simulink model "IEEE39_11gen"  (R2020a)
settings: Solver=FixedStepAuto  StartTime=0  StopTime=5  FixedStep=Ts  RelTol=1e-3
values from neighbouring files (symbols this model uses):
  Ts = 1/Fs    [ModifiedIEEE39_11gen.m]
  Wbase = Fbase*2*pi    [ModifiedIEEE39_11gen.m]
  Ybase = 1/Zbase    [ModifiedIEEE39_11gen.m]
  Zbase = Vbase/Ibase    [ModifiedIEEE39_11gen.m]
undefined symbols (not defined in the file or in its folder): ApparatusDiscreDamping, ApparatusPara, ApparatusPowerFlow, ApparatusType, OtherInputs, PowerFlow, x_e
libraries: powerlib x131, SimplusGT x51
settings Model: Creator=Qiufan_Yang  LastModifiedBy=Qiufan_Yang

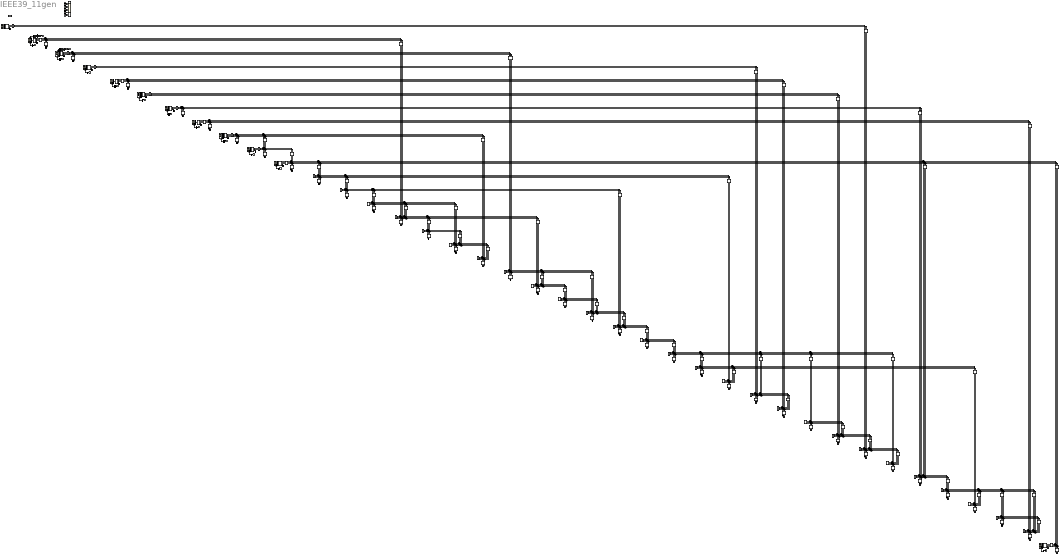
== system IEEE39_11gen ==
  B-GND{2,4,7,10,12,14,17,19,23,26,29,32,35,37,39..40,43,45,47,49,51,53,58,61..62,64..65,67,69,71..72,74,78..79,81..82} (36 alike) : powerlib/Elements/Ground  LConnTagsString=a
  Branch1-32 : powerlib/Elements/Three-Phase Series RLC Branch  LConnTagsString=A|B|C  RConnTagsString=A|B|C  BranchType=L  Resistance=(0)*Zbase  Inductance=(0.016321)*Zbase/Wbase  Capacitance=1e-6  Measurements=None
  Branch10-10 : powerlib/Elements/Three-Phase Parallel RLC Branch  LConnTagsString=A|B|C  RConnTagsString=A|B|C  BranchType=C  Resistance=(Inf)*Zbase  Inductance=(Inf)*Zbase/Wbase  Capacitance=(0.05)*Ybase/Wbase  Measurements=None
      settings: SourceProductBaseCode=PS
  Branch10-11 : powerlib/Elements/Three-Phase Series RLC Branch  LConnTagsString=A|B|C  RConnTagsString=A|B|C  BranchType=L  Resistance=(0)*Zbase  Inductance=(0.024661)*Zbase/Wbase  Capacitance=1e-6  Measurements=None
  Branch11-11 : powerlib/Elements/Three-Phase Parallel RLC Branch  LConnTagsString=A|B|C  RConnTagsString=A|B|C  BranchType=C  Resistance=(Inf)*Zbase  Inductance=(Inf)*Zbase/Wbase  Capacitance=(0.05)*Ybase/Wbase  Measurements=None
      settings: SourceProductBaseCode=PS
  Branch11-12 : powerlib/Elements/Three-Phase Series RLC Branch  LConnTagsString=A|B|C  RConnTagsString=A|B|C  BranchType=L  Resistance=(0)*Zbase  Inductance=(0.0090596)*Zbase/Wbase  Capacitance=1e-6  Measurements=None
  Branch11-34 : powerlib/Elements/Three-Phase Series RLC Branch  LConnTagsString=A|B|C  RConnTagsString=A|B|C  BranchType=L  Resistance=(0)*Zbase  Inductance=(0.00516)*Zbase/Wbase  Capacitance=1e-6  Measurements=None
  Branch11-39 : powerlib/Elements/Three-Phase Series RLC Branch  LConnTagsString=A|B|C  RConnTagsString=A|B|C  BranchType=L  Resistance=(0)*Zbase  Inductance=(0.01086)*Zbase/Wbase  Capacitance=1e-6  Measurements=None
  Branch12-12 : powerlib/Elements/Three-Phase Parallel RLC Branch  LConnTagsString=A|B|C  RConnTagsString=A|B|C  BranchType=C  Resistance=(Inf)*Zbase  Inductance=(Inf)*Zbase/Wbase  Capacitance=(0.03)*Ybase/Wbase  Measurements=None
      settings: SourceProductBaseCode=PS
  Branch12-13 : powerlib/Elements/Three-Phase Series RLC Branch  LConnTagsString=A|B|C  RConnTagsString=A|B|C  BranchType=L  Resistance=(0)*Zbase  Inductance=(0.01278)*Zbase/Wbase  Capacitance=1e-6  Measurements=None
  Branch12-27 : powerlib/Elements/Three-Phase Series RLC Branch  LConnTagsString=A|B|C  RConnTagsString=A|B|C  BranchType=L  Resistance=(0)*Zbase  Inductance=(0.0079802)*Zbase/Wbase  Capacitance=1e-6  Measurements=None
  Branch13-13 : powerlib/Elements/Three-Phase Parallel RLC Branch  LConnTagsString=A|B|C  RConnTagsString=A|B|C  BranchType=C  Resistance=(Inf)*Zbase  Inductance=(Inf)*Zbase/Wbase  Capacitance=(0.03)*Ybase/Wbase  Measurements=None
      settings: SourceProductBaseCode=PS
  Branch13-14 : powerlib/Elements/Three-Phase Series RLC Branch  LConnTagsString=A|B|C  RConnTagsString=A|B|C  BranchType=L  Resistance=(0)*Zbase  Inductance=(0.0076799)*Zbase/Wbase  Capacitance=1e-6  Measurements=None
  Branch13-23 : powerlib/Elements/Three-Phase Series RLC Branch  LConnTagsString=A|B|C  RConnTagsString=A|B|C  BranchType=L  Resistance=(0)*Zbase  Inductance=(0.0077399)*Zbase/Wbase  Capacitance=1e-6  Measurements=None
  Branch14-14 : powerlib/Elements/Three-Phase Parallel RLC Branch  LConnTagsString=A|B|C  RConnTagsString=A|B|C  BranchType=C  Resistance=(Inf)*Zbase  Inductance=(Inf)*Zbase/Wbase  Capacitance=(0.03)*Ybase/Wbase  Measurements=None
      settings: SourceProductBaseCode=PS
  Branch14-15 : powerlib/Elements/Three-Phase Series RLC Branch  LConnTagsString=A|B|C  RConnTagsString=A|B|C  BranchType=L  Resistance=(0)*Zbase  Inductance=(0.00156)*Zbase/Wbase  Capacitance=1e-6  Measurements=None
  Branch14-17 : powerlib/Elements/Three-Phase Series RLC Branch  LConnTagsString=A|B|C  RConnTagsString=A|B|C  BranchType=L  Resistance=(0)*Zbase  Inductance=(0.00672)*Zbase/Wbase  Capacitance=1e-6  Measurements=None
  Branch15-15 : powerlib/Elements/Three-Phase Parallel RLC Branch  LConnTagsString=A|B|C  RConnTagsString=A|B|C  BranchType=C  Resistance=(Inf)*Zbase  Inductance=(Inf)*Zbase/Wbase  Capacitance=(0.03)*Ybase/Wbase  Measurements=None
      settings: SourceProductBaseCode=PS
  Branch15-16 : powerlib/Elements/Three-Phase Series RLC Branch  LConnTagsString=A|B|C  RConnTagsString=A|B|C  BranchType=L  Resistance=(0)*Zbase  Inductance=(0.00552)*Zbase/Wbase  Capacitance=1e-6  Measurements=None
  Branch15-20 : powerlib/Elements/Three-Phase Series RLC Branch  LConnTagsString=A|B|C  RConnTagsString=A|B|C  BranchType=L  Resistance=(0)*Zbase  Inductance=(0.00492)*Zbase/Wbase  Capacitance=1e-6  Measurements=None
  Branch16-16 : powerlib/Elements/Three-Phase Parallel RLC Branch  LConnTagsString=A|B|C  RConnTagsString=A|B|C  BranchType=C  Resistance=(Inf)*Zbase  Inductance=(Inf)*Zbase/Wbase  Capacitance=(0.03)*Ybase/Wbase  Measurements=None
      settings: SourceProductBaseCode=PS
  Branch16-17 : powerlib/Elements/Three-Phase Series RLC Branch  LConnTagsString=A|B|C  RConnTagsString=A|B|C  BranchType=L  Resistance=(0)*Zbase  Inductance=(0.00276)*Zbase/Wbase  Capacitance=1e-6  Measurements=None
  Branch17-17 : powerlib/Elements/Three-Phase Parallel RLC Branch  LConnTagsString=A|B|C  RConnTagsString=A|B|C  BranchType=C  Resistance=(Inf)*Zbase  Inductance=(Inf)*Zbase/Wbase  Capacitance=(0.03)*Ybase/Wbase  Measurements=None
      settings: SourceProductBaseCode=PS
  Branch17-18 : powerlib/Elements/Three-Phase Series RLC Branch  LConnTagsString=A|B|C  RConnTagsString=A|B|C  BranchType=L  Resistance=(0)*Zbase  Inductance=(0.021782)*Zbase/Wbase  Capacitance=1e-6  Measurements=None
  Branch18-18 : powerlib/Elements/Three-Phase Parallel RLC Branch  LConnTagsString=A|B|C  RConnTagsString=A|B|C  BranchType=C  Resistance=(Inf)*Zbase  Inductance=(Inf)*Zbase/Wbase  Capacitance=(0.03)*Ybase/Wbase  Measurements=None
      settings: SourceProductBaseCode=PS
  Branch19-19 : powerlib/Elements/Three-Phase Parallel RLC Branch  LConnTagsString=A|B|C  RConnTagsString=A|B|C  BranchType=C  Resistance=(Inf)*Zbase  Inductance=(Inf)*Zbase/Wbase  Capacitance=(0.03)*Ybase/Wbase  Measurements=None
      settings: SourceProductBaseCode=PS
  Branch19-20 : powerlib/Elements/Three-Phase Series RLC Branch  LConnTagsString=A|B|C  RConnTagsString=A|B|C  BranchType=L  Resistance=(0)*Zbase  Inductance=(0.00258)*Zbase/Wbase  Capacitance=1e-6  Measurements=None
  Branch19-22 : powerlib/Elements/Three-Phase Series RLC Branch  LConnTagsString=A|B|C  RConnTagsString=A|B|C  BranchType=L  Resistance=(0)*Zbase  Inductance=(0.00258)*Zbase/Wbase  Capacitance=1e-6  Measurements=None
  Branch2-15 : powerlib/Elements/Three-Phase Series RLC Branch  LConnTagsString=A|B|C  RConnTagsString=A|B|C  BranchType=L  Resistance=(0)*Zbase  Inductance=(0.014999)*Zbase/Wbase  Capacitance=1e-6  Measurements=None
  Branch2-2 : powerlib/Elements/Three-Phase Parallel RLC Branch  LConnTagsString=A|B|C  RConnTagsString=A|B|C  BranchType=C  Resistance=(Inf)*Zbase  Inductance=(Inf)*Zbase/Wbase  Capacitance=(0.05)*Ybase/Wbase  Measurements=None
      settings: SourceProductBaseCode=PS
  Branch20-20 : powerlib/Elements/Three-Phase Parallel RLC Branch  LConnTagsString=A|B|C  RConnTagsString=A|B|C  BranchType=C  Resistance=(Inf)*Zbase  Inductance=(Inf)*Zbase/Wbase  Capacitance=(0.03)*Ybase/Wbase  Measurements=None
      settings: SourceProductBaseCode=PS
  Branch20-21 : powerlib/Elements/Three-Phase Series RLC Branch  LConnTagsString=A|B|C  RConnTagsString=A|B|C  BranchType=L  Resistance=(0)*Zbase  Inductance=(0.026103)*Zbase/Wbase  Capacitance=1e-6  Measurements=None
  Branch21-21 : powerlib/Elements/Three-Phase Parallel RLC Branch  LConnTagsString=A|B|C  RConnTagsString=A|B|C  BranchType=C  Resistance=(Inf)*Zbase  Inductance=(Inf)*Zbase/Wbase  Capacitance=(0.03)*Ybase/Wbase  Measurements=None
      settings: SourceProductBaseCode=PS
  Branch21-22 : powerlib/Elements/Three-Phase Series RLC Branch  LConnTagsString=A|B|C  RConnTagsString=A|B|C  BranchType=L  Resistance=(0)*Zbase  Inductance=(0.026103)*Zbase/Wbase  Capacitance=1e-6  Measurements=None
  Branch22-22 : powerlib/Elements/Three-Phase Parallel RLC Branch  LConnTagsString=A|B|C  RConnTagsString=A|B|C  BranchType=C  Resistance=(Inf)*Zbase  Inductance=(Inf)*Zbase/Wbase  Capacitance=(0.03)*Ybase/Wbase  Measurements=None
      settings: SourceProductBaseCode=PS
  Branch22-23 : powerlib/Elements/Three-Phase Series RLC Branch  LConnTagsString=A|B|C  RConnTagsString=A|B|C  BranchType=L  Resistance=(0)*Zbase  Inductance=(0.0060599)*Zbase/Wbase  Capacitance=1e-6  Measurements=None
  Branch23-23 : powerlib/Elements/Three-Phase Parallel RLC Branch  LConnTagsString=A|B|C  RConnTagsString=A|B|C  BranchType=C  Resistance=(Inf)*Zbase  Inductance=(Inf)*Zbase/Wbase  Capacitance=(0.03)*Ybase/Wbase  Measurements=None
      settings: SourceProductBaseCode=PS
  Branch23-24 : powerlib/Elements/Three-Phase Series RLC Branch  LConnTagsString=A|B|C  RConnTagsString=A|B|C  BranchType=L  Resistance=(0)*Zbase  Inductance=(0.013021)*Zbase/Wbase  Capacitance=1e-6  Measurements=None
  Branch24-24 : powerlib/Elements/Three-Phase Parallel RLC Branch  LConnTagsString=A|B|C  RConnTagsString=A|B|C  BranchType=C  Resistance=(Inf)*Zbase  Inductance=(Inf)*Zbase/Wbase  Capacitance=(0.03)*Ybase/Wbase  Measurements=None
      settings: SourceProductBaseCode=PS
  Branch24-25 : powerlib/Elements/Three-Phase Series RLC Branch  LConnTagsString=A|B|C  RConnTagsString=A|B|C  BranchType=L  Resistance=(0)*Zbase  Inductance=(0.0056398)*Zbase/Wbase  Capacitance=1e-6  Measurements=None
  Branch25-25 : powerlib/Elements/Three-Phase Parallel RLC Branch  LConnTagsString=A|B|C  RConnTagsString=A|B|C  BranchType=C  Resistance=(Inf)*Zbase  Inductance=(Inf)*Zbase/Wbase  Capacitance=(0.03)*Ybase/Wbase  Measurements=None
      settings: SourceProductBaseCode=PS
  Branch25-26 : powerlib/Elements/Three-Phase Series RLC Branch  LConnTagsString=A|B|C  RConnTagsString=A|B|C  BranchType=L  Resistance=(0)*Zbase  Inductance=(0.0053399)*Zbase/Wbase  Capacitance=1e-6  Measurements=None
  Branch25-28 : powerlib/Elements/Three-Phase Series RLC Branch  LConnTagsString=A|B|C  RConnTagsString=A|B|C  BranchType=L  Resistance=(0)*Zbase  Inductance=(0.0117)*Zbase/Wbase  Capacitance=1e-6  Measurements=None
  Branch25-30 : powerlib/Elements/Three-Phase Series RLC Branch  LConnTagsString=A|B|C  RConnTagsString=A|B|C  BranchType=L  Resistance=(0)*Zbase  Inductance=(0.0080998)*Zbase/Wbase  Capacitance=1e-6  Measurements=None
  Branch25-33 : powerlib/Elements/Three-Phase Series RLC Branch  LConnTagsString=A|B|C  RConnTagsString=A|B|C  BranchType=L  Resistance=(0)*Zbase  Inductance=(0.0035399)*Zbase/Wbase  Capacitance=1e-6  Measurements=None
  Branch26-26 : powerlib/Elements/Three-Phase Parallel RLC Branch  LConnTagsString=A|B|C  RConnTagsString=A|B|C  BranchType=C  Resistance=(Inf)*Zbase  Inductance=(Inf)*Zbase/Wbase  Capacitance=(0.03)*Ybase/Wbase  Measurements=None
      settings: SourceProductBaseCode=PS
  Branch26-27 : powerlib/Elements/Three-Phase Series RLC Branch  LConnTagsString=A|B|C  RConnTagsString=A|B|C  BranchType=L  Resistance=(0)*Zbase  Inductance=(0.00492)*Zbase/Wbase  Capacitance=1e-6  Measurements=None
  Branch26-36 : powerlib/Elements/Three-Phase Series RLC Branch  LConnTagsString=A|B|C  RConnTagsString=A|B|C  BranchType=L  Resistance=(0)*Zbase  Inductance=(0.01038)*Zbase/Wbase  Capacitance=1e-6  Measurements=None
  Branch27-27 : powerlib/Elements/Three-Phase Parallel RLC Branch  LConnTagsString=A|B|C  RConnTagsString=A|B|C  BranchType=C  Resistance=(Inf)*Zbase  Inductance=(Inf)*Zbase/Wbase  Capacitance=(0.03)*Ybase/Wbase  Measurements=None
      settings: SourceProductBaseCode=PS
  Branch28-28 : powerlib/Elements/Three-Phase Parallel RLC Branch  LConnTagsString=A|B|C  RConnTagsString=A|B|C  BranchType=C  Resistance=(Inf)*Zbase  Inductance=(Inf)*Zbase/Wbase  Capacitance=(0.03)*Ybase/Wbase  Measurements=None
      settings: SourceProductBaseCode=PS
  Branch28-29 : powerlib/Elements/Three-Phase Series RLC Branch  LConnTagsString=A|B|C  RConnTagsString=A|B|C  BranchType=L  Resistance=(0)*Zbase  Inductance=(0.0082802)*Zbase/Wbase  Capacitance=1e-6  Measurements=None
  Branch29-29 : powerlib/Elements/Three-Phase Parallel RLC Branch  LConnTagsString=A|B|C  RConnTagsString=A|B|C  BranchType=C  Resistance=(Inf)*Zbase  Inductance=(Inf)*Zbase/Wbase  Capacitance=(0.03)*Ybase/Wbase  Measurements=None
      settings: SourceProductBaseCode=PS
  Branch3-19 : powerlib/Elements/Three-Phase Series RLC Branch  LConnTagsString=A|B|C  RConnTagsString=A|B|C  BranchType=L  Resistance=(0)*Zbase  Inductance=(0.012)*Zbase/Wbase  Capacitance=1e-6  Measurements=None
  Branch3-3 : powerlib/Elements/Three-Phase Parallel RLC Branch  LConnTagsString=A|B|C  RConnTagsString=A|B|C  BranchType=C  Resistance=(Inf)*Zbase  Inductance=(Inf)*Zbase/Wbase  Capacitance=(0.05)*Ybase/Wbase  Measurements=None
      settings: SourceProductBaseCode=PS
  Branch30-30 : powerlib/Elements/Three-Phase Parallel RLC Branch  LConnTagsString=A|B|C  RConnTagsString=A|B|C  BranchType=C  Resistance=(Inf)*Zbase  Inductance=(Inf)*Zbase/Wbase  Capacitance=(0.03)*Ybase/Wbase  Measurements=None
      settings: SourceProductBaseCode=PS
  Branch30-31 : powerlib/Elements/Three-Phase Series RLC Branch  LConnTagsString=A|B|C  RConnTagsString=A|B|C  BranchType=L  Resistance=(0)*Zbase  Inductance=(0.0083998)*Zbase/Wbase  Capacitance=1e-6  Measurements=None
  Branch31-31 : powerlib/Elements/Three-Phase Parallel RLC Branch  LConnTagsString=A|B|C  RConnTagsString=A|B|C  BranchType=C  Resistance=(Inf)*Zbase  Inductance=(Inf)*Zbase/Wbase  Capacitance=(0.03)*Ybase/Wbase  Measurements=None
      settings: SourceProductBaseCode=PS
  Branch31-32 : powerlib/Elements/Three-Phase Series RLC Branch  LConnTagsString=A|B|C  RConnTagsString=A|B|C  BranchType=L  Resistance=(0)*Zbase  Inductance=(0.00576)*Zbase/Wbase  Capacitance=1e-6  Measurements=None
  Branch32-32 : powerlib/Elements/Three-Phase Parallel RLC Branch  LConnTagsString=A|B|C  RConnTagsString=A|B|C  BranchType=C  Resistance=(Inf)*Zbase  Inductance=(Inf)*Zbase/Wbase  Capacitance=(0.03)*Ybase/Wbase  Measurements=None
      settings: SourceProductBaseCode=PS
  Branch32-33 : powerlib/Elements/Three-Phase Series RLC Branch  LConnTagsString=A|B|C  RConnTagsString=A|B|C  BranchType=L  Resistance=(0)*Zbase  Inductance=(0.021)*Zbase/Wbase  Capacitance=1e-6  Measurements=None
  Branch33-33 : powerlib/Elements/Three-Phase Parallel RLC Branch  LConnTagsString=A|B|C  RConnTagsString=A|B|C  BranchType=C  Resistance=(Inf)*Zbase  Inductance=(Inf)*Zbase/Wbase  Capacitance=(0.03)*Ybase/Wbase  Measurements=None
      settings: SourceProductBaseCode=PS
  Branch34-34 : powerlib/Elements/Three-Phase Parallel RLC Branch  LConnTagsString=A|B|C  RConnTagsString=A|B|C  BranchType=C  Resistance=(Inf)*Zbase  Inductance=(Inf)*Zbase/Wbase  Capacitance=(0.03)*Ybase/Wbase  Measurements=None
      settings: SourceProductBaseCode=PS
  Branch34-35 : powerlib/Elements/Three-Phase Series RLC Branch  LConnTagsString=A|B|C  RConnTagsString=A|B|C  BranchType=L  Resistance=(0)*Zbase  Inductance=(0.019011)*Zbase/Wbase  Capacitance=1e-6  Measurements=None
  Branch35-35 : powerlib/Elements/Three-Phase Parallel RLC Branch  LConnTagsString=A|B|C  RConnTagsString=A|B|C  BranchType=C  Resistance=(Inf)*Zbase  Inductance=(Inf)*Zbase/Wbase  Capacitance=(0.03)*Ybase/Wbase  Measurements=None
      settings: SourceProductBaseCode=PS
  Branch35-36 : powerlib/Elements/Three-Phase Series RLC Branch  LConnTagsString=A|B|C  RConnTagsString=A|B|C  BranchType=L  Resistance=(0)*Zbase  Inductance=(0.0088199)*Zbase/Wbase  Capacitance=1e-6  Measurements=None
  Branch35-37 : powerlib/Elements/Three-Phase Series RLC Branch  LConnTagsString=A|B|C  RConnTagsString=A|B|C  BranchType=L  Resistance=(0)*Zbase  Inductance=(0.028441)*Zbase/Wbase  Capacitance=1e-6  Measurements=None
  Branch35-38 : powerlib/Elements/Three-Phase Series RLC Branch  LConnTagsString=A|B|C  RConnTagsString=A|B|C  BranchType=L  Resistance=(0)*Zbase  Inductance=(0.037495)*Zbase/Wbase  Capacitance=1e-6  Measurements=None
  Branch36-36 : powerlib/Elements/Three-Phase Parallel RLC Branch  LConnTagsString=A|B|C  RConnTagsString=A|B|C  BranchType=C  Resistance=(Inf)*Zbase  Inductance=(Inf)*Zbase/Wbase  Capacitance=(0.03)*Ybase/Wbase  Measurements=None
      settings: SourceProductBaseCode=PS
  Branch37-37 : powerlib/Elements/Three-Phase Parallel RLC Branch  LConnTagsString=A|B|C  RConnTagsString=A|B|C  BranchType=C  Resistance=(Inf)*Zbase  Inductance=(Inf)*Zbase/Wbase  Capacitance=(0.03)*Ybase/Wbase  Measurements=None
      settings: SourceProductBaseCode=PS
  Branch37-38 : powerlib/Elements/Three-Phase Series RLC Branch  LConnTagsString=A|B|C  RConnTagsString=A|B|C  BranchType=L  Resistance=(0)*Zbase  Inductance=(0.0090596)*Zbase/Wbase  Capacitance=1e-6  Measurements=None
  Branch38-38 : powerlib/Elements/Three-Phase Parallel RLC Branch  LConnTagsString=A|B|C  RConnTagsString=A|B|C  BranchType=C  Resistance=(Inf)*Zbase  Inductance=(Inf)*Zbase/Wbase  Capacitance=(0.03)*Ybase/Wbase  Measurements=None
      settings: SourceProductBaseCode=PS
  Branch39-39 : powerlib/Elements/Three-Phase Parallel RLC Branch  LConnTagsString=A|B|C  RConnTagsString=A|B|C  BranchType=C  Resistance=(Inf)*Zbase  Inductance=(Inf)*Zbase/Wbase  Capacitance=(0.05)*Ybase/Wbase  Measurements=None
      settings: SourceProductBaseCode=PS
  Branch4-28 : powerlib/Elements/Three-Phase Series RLC Branch  LConnTagsString=A|B|C  RConnTagsString=A|B|C  BranchType=L  Resistance=(0)*Zbase  Inductance=(0.0085201)*Zbase/Wbase  Capacitance=1e-6  Measurements=None
  Branch5-29 : powerlib/Elements/Three-Phase Series RLC Branch  LConnTagsString=A|B|C  RConnTagsString=A|B|C  BranchType=L  Resistance=(0)*Zbase  Inductance=(0.0108)*Zbase/Wbase  Capacitance=1e-6  Measurements=None
  Branch5-5 : powerlib/Elements/Three-Phase Parallel RLC Branch  LConnTagsString=A|B|C  RConnTagsString=A|B|C  BranchType=C  Resistance=(Inf)*Zbase  Inductance=(Inf)*Zbase/Wbase  Capacitance=(0.05)*Ybase/Wbase  Measurements=None
      settings: SourceProductBaseCode=PS
  Branch6-31 : powerlib/Elements/Three-Phase Series RLC Branch  LConnTagsString=A|B|C  RConnTagsString=A|B|C  BranchType=L  Resistance=(0)*Zbase  Inductance=(0.00858)*Zbase/Wbase  Capacitance=1e-6  Measurements=None
  Branch7-34 : powerlib/Elements/Three-Phase Series RLC Branch  LConnTagsString=A|B|C  RConnTagsString=A|B|C  BranchType=L  Resistance=(0)*Zbase  Inductance=(0.01392)*Zbase/Wbase  Capacitance=1e-6  Measurements=None
  Branch7-7 : powerlib/Elements/Three-Phase Parallel RLC Branch  LConnTagsString=A|B|C  RConnTagsString=A|B|C  BranchType=C  Resistance=(Inf)*Zbase  Inductance=(Inf)*Zbase/Wbase  Capacitance=(0.05)*Ybase/Wbase  Measurements=None
      settings: SourceProductBaseCode=PS
  Branch8-38 : powerlib/Elements/Three-Phase Series RLC Branch  LConnTagsString=A|B|C  RConnTagsString=A|B|C  BranchType=L  Resistance=(0)*Zbase  Inductance=(0.0093598)*Zbase/Wbase  Capacitance=1e-6  Measurements=None
  Branch8-8 : powerlib/Elements/Three-Phase Parallel RLC Branch  LConnTagsString=A|B|C  RConnTagsString=A|B|C  BranchType=C  Resistance=(Inf)*Zbase  Inductance=(Inf)*Zbase/Wbase  Capacitance=(0.05)*Ybase/Wbase  Measurements=None
      settings: SourceProductBaseCode=PS
  Branch9-10 : powerlib/Elements/Three-Phase Series RLC Branch  LConnTagsString=A|B|C  RConnTagsString=A|B|C  BranchType=L  Resistance=(0)*Zbase  Inductance=(0.014999)*Zbase/Wbase  Capacitance=1e-6  Measurements=None
  Branch9-18 : powerlib/Elements/Three-Phase Series RLC Branch  LConnTagsString=A|B|C  RConnTagsString=A|B|C  BranchType=L  Resistance=(0)*Zbase  Inductance=(0.014999)*Zbase/Wbase  Capacitance=1e-6  Measurements=None
  Branch9-9 : powerlib/Elements/Three-Phase Parallel RLC Branch  LConnTagsString=A|B|C  RConnTagsString=A|B|C  BranchType=C  Resistance=(Inf)*Zbase  Inductance=(Inf)*Zbase/Wbase  Capacitance=(0.05)*Ybase/Wbase  Measurements=None
      settings: SourceProductBaseCode=PS
  Bus{1..39} (39 alike) : SimplusGT/Three-Phase Bus  Vbase=1  Sbase=1
      settings: SourceProductName=Simplus Grid Tool
  D-GND{1..11,39} (12 alike) : powerlib/Elements/Ground  LConnTagsString=a
  D-Scope{1..11,39} (12 alike) : Scope  NumInputPorts=7
  DS-Bus{1..11,39} (12 alike) : BusSelector  OutputSignals=v_dq,i_dq,v_abc,i_abc,w,theta,pq
  Demux{1..13} (13 alike) : Demux  Outputs=2
  Inf-Bus1 : SimplusGT/AC Infinite Bus (Voltage Type)  Ts=Ts  Sbase=Sbase  Vbase=Vbase  Wbase=Wbase  vd=PowerFlow{1}(3)  vq=0  theta0=PowerFlow{1}(4)  w=Wbase  R=1e-30
      settings: SourceProductName=Simplus Grid Tool
  Scope1 : Scope  NumInputPorts=9
  Sqrt1 : Sqrt  SaturateOnIntegerOverflow=on
  Sqrt2 : Sqrt  SaturateOnIntegerOverflow=on
  Square{2..5} (4 alike) : Math  Operator=square  SaturateOnIntegerOverflow=on
  Sum1 : Sum  Inputs=|++
  Sum2 : Sum  Inputs=|++
  VSI-Droop4 : SimplusGT/Grid-Forming Voltage-Source Inverter (dq-Frame System Object)  Ts=Ts  Sbase=Sbase  Vbase=Vbase  Wbase=Wbase  ApparatusType=ApparatusType{4}  ApparatusPara=ApparatusPara{4}  PowerFlow=ApparatusPowerFlow{4}  x0=x_e{4}  OtherInputs=OtherInputs{4}  DiscreMethod=Hybrid Trapezoidal  EnableInsideModification=off  DiscreDampingFlag=on  DiscreDampingValue=ApparatusDiscreDamping{4}  LinearizationTimes=1  DirectFeedthrough=off
      settings: SourceProductName=Simplus Grid Tool
  VSI-Droop6 : SimplusGT/Grid-Forming Voltage-Source Inverter (dq-Frame System Object)  Ts=Ts  Sbase=Sbase  Vbase=Vbase  Wbase=Wbase  ApparatusType=ApparatusType{6}  ApparatusPara=ApparatusPara{6}  PowerFlow=ApparatusPowerFlow{6}  x0=x_e{6}  OtherInputs=OtherInputs{6}  DiscreMethod=Hybrid Trapezoidal  EnableInsideModification=off  DiscreDampingFlag=on  DiscreDampingValue=ApparatusDiscreDamping{6}  LinearizationTimes=1  DirectFeedthrough=off
      settings: SourceProductName=Simplus Grid Tool
  VSI-PLL10 : SimplusGT/Grid-Following Voltage-Source Inverter (dq-Frame System Object)  Ts=Ts  Sbase=Sbase  Vbase=Vbase  Wbase=Wbase  ApparatusType=ApparatusType{10}  ApparatusPara=ApparatusPara{10}  PowerFlow=ApparatusPowerFlow{10}  x0=x_e{10}  OtherInputs=OtherInputs{10}  DiscreMethod=Hybrid Trapezoidal  EnableInsideModification=off  DiscreDampingFlag=on  DiscreDampingValue=ApparatusDiscreDamping{10}  LinearizationTimes=1  DirectFeedthrough=off
      settings: SourceProductName=Simplus Grid Tool
  VSI-PLL11 : SimplusGT/Grid-Following Voltage-Source Inverter (dq-Frame System Object)  Ts=Ts  Sbase=Sbase  Vbase=Vbase  Wbase=Wbase  ApparatusType=ApparatusType{11}  ApparatusPara=ApparatusPara{11}  PowerFlow=ApparatusPowerFlow{11}  x0=x_e{11}  OtherInputs=OtherInputs{11}  DiscreMethod=Hybrid Trapezoidal  EnableInsideModification=off  DiscreDampingFlag=on  DiscreDampingValue=ApparatusDiscreDamping{11}  LinearizationTimes=1  DirectFeedthrough=off
      settings: SourceProductName=Simplus Grid Tool
  VSI-PLL2 : SimplusGT/Grid-Following Voltage-Source Inverter (dq-Frame System Object)  Ts=Ts  Sbase=Sbase  Vbase=Vbase  Wbase=Wbase  ApparatusType=ApparatusType{2}  ApparatusPara=ApparatusPara{2}  PowerFlow=ApparatusPowerFlow{2}  x0=x_e{2}  OtherInputs=OtherInputs{2}  DiscreMethod=Hybrid Trapezoidal  EnableInsideModification=off  DiscreDampingFlag=on  DiscreDampingValue=ApparatusDiscreDamping{2}  LinearizationTimes=1  DirectFeedthrough=off
      settings: SourceProductName=Simplus Grid Tool
  VSI-PLL3 : SimplusGT/Grid-Following Voltage-Source Inverter (dq-Frame System Object)  Ts=Ts  Sbase=Sbase  Vbase=Vbase  Wbase=Wbase  ApparatusType=ApparatusType{3}  ApparatusPara=ApparatusPara{3}  PowerFlow=ApparatusPowerFlow{3}  x0=x_e{3}  OtherInputs=OtherInputs{3}  DiscreMethod=Hybrid Trapezoidal  EnableInsideModification=off  DiscreDampingFlag=on  DiscreDampingValue=ApparatusDiscreDamping{3}  LinearizationTimes=1  DirectFeedthrough=off
      settings: SourceProductName=Simplus Grid Tool
  VSI-PLL39 : SimplusGT/Grid-Following Voltage-Source Inverter (dq-Frame System Object)  Ts=Ts  Sbase=Sbase  Vbase=Vbase  Wbase=Wbase  ApparatusType=ApparatusType{39}  ApparatusPara=ApparatusPara{39}  PowerFlow=ApparatusPowerFlow{39}  x0=x_e{39}  OtherInputs=OtherInputs{39}  DiscreMethod=Hybrid Trapezoidal  EnableInsideModification=off  DiscreDampingFlag=on  DiscreDampingValue=ApparatusDiscreDamping{39}  LinearizationTimes=1  DirectFeedthrough=off
      settings: SourceProductName=Simplus Grid Tool
  VSI-PLL5 : SimplusGT/Grid-Following Voltage-Source Inverter (dq-Frame System Object)  Ts=Ts  Sbase=Sbase  Vbase=Vbase  Wbase=Wbase  ApparatusType=ApparatusType{5}  ApparatusPara=ApparatusPara{5}  PowerFlow=ApparatusPowerFlow{5}  x0=x_e{5}  OtherInputs=OtherInputs{5}  DiscreMethod=Hybrid Trapezoidal  EnableInsideModification=off  DiscreDampingFlag=on  DiscreDampingValue=ApparatusDiscreDamping{5}  LinearizationTimes=1  DirectFeedthrough=off
      settings: SourceProductName=Simplus Grid Tool
  VSI-PLL7 : SimplusGT/Grid-Following Voltage-Source Inverter (dq-Frame System Object)  Ts=Ts  Sbase=Sbase  Vbase=Vbase  Wbase=Wbase  ApparatusType=ApparatusType{7}  ApparatusPara=ApparatusPara{7}  PowerFlow=ApparatusPowerFlow{7}  x0=x_e{7}  OtherInputs=OtherInputs{7}  DiscreMethod=Hybrid Trapezoidal  EnableInsideModification=off  DiscreDampingFlag=on  DiscreDampingValue=ApparatusDiscreDamping{7}  LinearizationTimes=1  DirectFeedthrough=off
      settings: SourceProductName=Simplus Grid Tool
  VSI-PLL8 : SimplusGT/Grid-Following Voltage-Source Inverter (dq-Frame System Object)  Ts=Ts  Sbase=Sbase  Vbase=Vbase  Wbase=Wbase  ApparatusType=ApparatusType{8}  ApparatusPara=ApparatusPara{8}  PowerFlow=ApparatusPowerFlow{8}  x0=x_e{8}  OtherInputs=OtherInputs{8}  DiscreMethod=Hybrid Trapezoidal  EnableInsideModification=off  DiscreDampingFlag=on  DiscreDampingValue=ApparatusDiscreDamping{8}  LinearizationTimes=1  DirectFeedthrough=off
      settings: SourceProductName=Simplus Grid Tool
  VSI-PLL9 : SimplusGT/Grid-Following Voltage-Source Inverter (dq-Frame System Object)  Ts=Ts  Sbase=Sbase  Vbase=Vbase  Wbase=Wbase  ApparatusType=ApparatusType{9}  ApparatusPara=ApparatusPara{9}  PowerFlow=ApparatusPowerFlow{9}  x0=x_e{9}  OtherInputs=OtherInputs{9}  DiscreMethod=Hybrid Trapezoidal  EnableInsideModification=off  DiscreDampingFlag=on  DiscreDampingValue=ApparatusDiscreDamping{9}  LinearizationTimes=1  DirectFeedthrough=off
      settings: SourceProductName=Simplus Grid Tool
  powergui : powerlib/powergui  Priority=1  SimulationMode=Discrete  SampleTime=Ts  frequency=60  Iterations=50  frequencyindice=0  Pbase=100e6  ErrMax=1e-4  UnitsV=kV  UnitsW=MW  buscounter=0  FunctionMessages=off  echomessages=off  EnableUseOfTLC=off  CurrentSourceSwitches=off  DisableSnubberDevices=off  DisableRonSwitches=off  DisableVfSwitches=off  DisplayEquations=off  AutomaticDiscreteSolvers=off  SolverType=Tustin/Backward Euler (TBE)  Interpol=off  ExternalGateDelay=off  methode=off  Ts=100  x0status=blocks  SPID=on  SwTol=0  HookPort=off  NonlinearTolerance=1e-4  nMaxIteration=100  ContinueOnMaxIteration=off  RestoreLinks=warning  ResistiveCurrentMeasurement=off  Frange=[0:2:500]  Ylog=off  Xlog=on  ShowGrid=off  save=off  variable=ZData  structure=0  ZoomFFT=off  StartTime=0.0  cycles=1  DisplayStyle=1  fundamental=60  FreqAxis=off  MaxFrequency=1000  frequencyindicesteady=1  RmsSteady=1  display=off
  wires:
  Inf-Bus1/1 -> DS-Bus1/1
  DS-Bus1/1 -> D-Scope1/1  "<v_dq>"
  DS-Bus1/2 -> D-Scope1/2  "<i_dq>"
  DS-Bus1/3 -> D-Scope1/3  "<v_abc>"
  DS-Bus1/4 -> D-Scope1/4  "<i_abc>"
  DS-Bus1/5 -> D-Scope1/5  "<w>"
  DS-Bus1/6 -> D-Scope1/6  "<theta>"
  DS-Bus1/7 -> D-Scope1/7  "<pq>"
  VSI-PLL2/1 -> DS-Bus2/1
  DS-Bus2/2 -> D-Scope2/2  "<i_dq>"
  DS-Bus2/3 -> D-Scope2/3  "<v_abc>"
  DS-Bus2/4 -> D-Scope2/4  "<i_abc>"
  DS-Bus2/5 -> D-Scope2/5  "<w>"
  DS-Bus2/6 -> D-Scope2/6  "<theta>"
  VSI-PLL3/1 -> DS-Bus3/1
  DS-Bus3/2 -> D-Scope3/2  "<i_dq>"
  DS-Bus3/3 -> D-Scope3/3  "<v_abc>"
  DS-Bus3/4 -> D-Scope3/4  "<i_abc>"
  DS-Bus3/5 -> D-Scope3/5  "<w>"
  DS-Bus3/6 -> D-Scope3/6  "<theta>"
  VSI-Droop4/1 -> DS-Bus4/1
  DS-Bus4/1 -> D-Scope4/1  "<v_dq>"
  DS-Bus4/2 -> D-Scope4/2  "<i_dq>"
  DS-Bus4/3 -> D-Scope4/3  "<v_abc>"
  DS-Bus4/4 -> D-Scope4/4  "<i_abc>"
  DS-Bus4/5 -> D-Scope4/5  "<w>"
  DS-Bus4/6 -> D-Scope4/6  "<theta>"
  VSI-PLL5/1 -> DS-Bus5/1
  DS-Bus5/1 -> D-Scope5/1  "<v_dq>"
  DS-Bus5/2 -> D-Scope5/2  "<i_dq>"
  DS-Bus5/3 -> D-Scope5/3  "<v_abc>"
  DS-Bus5/4 -> D-Scope5/4  "<i_abc>"
  DS-Bus5/5 -> D-Scope5/5  "<w>"
  DS-Bus5/6 -> D-Scope5/6  "<theta>"
  VSI-Droop6/1 -> DS-Bus6/1
  DS-Bus6/1 -> D-Scope6/1  "<v_dq>"
  DS-Bus6/2 -> D-Scope6/2  "<i_dq>"
  DS-Bus6/3 -> D-Scope6/3  "<v_abc>"
  DS-Bus6/4 -> D-Scope6/4  "<i_abc>"
  DS-Bus6/5 -> D-Scope6/5  "<w>"
  DS-Bus6/6 -> D-Scope6/6  "<theta>"
  VSI-PLL7/1 -> DS-Bus7/1
  DS-Bus7/1 -> D-Scope7/1  "<v_dq>"
  DS-Bus7/2 -> D-Scope7/2  "<i_dq>"
  DS-Bus7/3 -> D-Scope7/3  "<v_abc>"
  DS-Bus7/4 -> D-Scope7/4  "<i_abc>"
  DS-Bus7/5 -> D-Scope7/5  "<w>"
  DS-Bus7/6 -> D-Scope7/6  "<theta>"
  VSI-PLL8/1 -> DS-Bus8/1
  DS-Bus8/1 -> D-Scope8/1  "<v_dq>"
  DS-Bus8/2 -> D-Scope8/2  "<i_dq>"
  DS-Bus8/3 -> D-Scope8/3  "<v_abc>"
  DS-Bus8/4 -> D-Scope8/4  "<i_abc>"
  DS-Bus8/5 -> D-Scope8/5  "<w>"
  DS-Bus8/6 -> D-Scope8/6  "<theta>"
  VSI-PLL9/1 -> DS-Bus9/1
  DS-Bus9/1 -> D-Scope9/1  "<v_dq>"
  DS-Bus9/2 -> D-Scope9/2  "<i_dq>"
  DS-Bus9/3 -> D-Scope9/3  "<v_abc>"
  DS-Bus9/4 -> D-Scope9/4  "<i_abc>"
  DS-Bus9/5 -> D-Scope9/5  "<w>"
  DS-Bus9/6 -> D-Scope9/6  "<theta>"
  VSI-PLL10/1 -> DS-Bus10/1
  DS-Bus10/1 -> D-Scope10/1  "<v_dq>"
  DS-Bus10/2 -> D-Scope10/2  "<i_dq>"
  DS-Bus10/3 -> D-Scope10/3  "<v_abc>"
  DS-Bus10/4 -> D-Scope10/4  "<i_abc>"
  DS-Bus10/5 -> D-Scope10/5  "<w>"
  DS-Bus10/6 -> D-Scope10/6  "<theta>"
  VSI-PLL11/1 -> DS-Bus11/1
  DS-Bus11/1 -> D-Scope11/1  "<v_dq>"
  DS-Bus11/2 -> D-Scope11/2  "<i_dq>"
  DS-Bus11/3 -> D-Scope11/3  "<v_abc>"
  DS-Bus11/4 -> D-Scope11/4  "<i_abc>"
  DS-Bus11/5 -> D-Scope11/5  "<w>"
  DS-Bus11/6 -> D-Scope11/6  "<theta>"
  VSI-PLL39/1 -> DS-Bus39/1
  DS-Bus39/1 -> D-Scope39/1  "<v_dq>"
  DS-Bus39/2 -> D-Scope39/2  "<i_dq>"
  DS-Bus39/3 -> D-Scope39/3  "<v_abc>"
  DS-Bus39/4 -> D-Scope39/4  "<i_abc>"
  DS-Bus39/5 -> D-Scope39/5  "<w>"
  DS-Bus39/6 -> D-Scope39/6  "<theta>"
  Demux1/1 -> Square2/1
  Square2/1 -> Sum1/1
  DS-Bus2/1 -> Demux1/1, D-Scope2/1  "<v_dq>"
  Sqrt1/1 -> [u2]
  Sum1/1 -> Sqrt1/1
  Square3/1 -> Sum1/2
  Demux1/2 -> Square3/1
  DS-Bus3/1 -> Demux2/1, D-Scope3/1  "<v_dq>"
  Square5/1 -> Sum2/2
  Sqrt2/1 -> [u3]
  Square4/1 -> Sum2/1
  Demux2/2 -> Square5/1
  Demux2/1 -> Square4/1
  Sum2/1 -> Sqrt2/1
  Demux11/1 -> [p2]
  DS-Bus2/7 -> Demux11/1, D-Scope2/7  "<pq>"
  Demux3/1 -> [p3]
  DS-Bus3/7 -> Demux3/1, D-Scope3/7  "<pq>"
  Demux4/1 -> [p4]
  DS-Bus4/7 -> Demux4/1, D-Scope4/7  "<pq>"
  Demux5/1 -> [p5]
  DS-Bus5/7 -> Demux5/1, D-Scope5/7  "<pq>"
  Demux6/1 -> [p6]
  DS-Bus6/7 -> Demux6/1, D-Scope6/7  "<pq>"
  Demux7/1 -> [p7]
  DS-Bus7/7 -> Demux7/1, D-Scope7/7  "<pq>"
  Demux8/1 -> [p8]
  DS-Bus8/7 -> Demux8/1, D-Scope8/7  "<pq>"
  Demux9/1 -> [p9]
  DS-Bus9/7 -> Demux9/1, D-Scope9/7  "<pq>"
  Demux10/1 -> [p10]
  DS-Bus10/7 -> Demux10/1, D-Scope10/7  "<pq>"
  Demux12/1 -> [p11]
  DS-Bus11/7 -> Demux12/1, D-Scope11/7  "<pq>"
  Demux13/1 -> [p1]
  DS-Bus39/7 -> Demux13/1, D-Scope39/7  "<pq>"
  [p2] -> Scope1/2
  [p9] -> Scope1/7
  [p7] -> Scope1/5
  [p3] -> Scope1/3
  [p1] -> Scope1/1
  [p10] -> Scope1/8
  [p5] -> Scope1/4
  [p8] -> Scope1/6
  [p11] -> Scope1/9
  connections:
  Inf-Bus1/LConn4 -- D-GND1/LConn1
  VSI-PLL2/LConn4 -- D-GND2/LConn1
  VSI-PLL3/LConn4 -- D-GND3/LConn1
  VSI-Droop4/LConn4 -- D-GND4/LConn1
  VSI-PLL5/LConn4 -- D-GND5/LConn1
  VSI-Droop6/LConn4 -- D-GND6/LConn1
  VSI-PLL7/LConn4 -- D-GND7/LConn1
  VSI-PLL8/LConn4 -- D-GND8/LConn1
  VSI-PLL9/LConn4 -- D-GND9/LConn1
  VSI-PLL10/LConn4 -- D-GND10/LConn1
  VSI-PLL11/LConn4 -- D-GND11/LConn1
  VSI-PLL39/LConn4 -- D-GND39/LConn1
  Branch2-2/RConn1 -- Branch2-2/RConn2 -- Branch2-2/RConn3 -- B-GND2/LConn1
  Branch3-3/RConn1 -- Branch3-3/RConn2 -- Branch3-3/RConn3 -- B-GND4/LConn1
  Branch5-5/RConn1 -- Branch5-5/RConn2 -- Branch5-5/RConn3 -- B-GND7/LConn1
  Branch7-7/RConn1 -- Branch7-7/RConn2 -- Branch7-7/RConn3 -- B-GND10/LConn1
  Branch8-8/RConn1 -- Branch8-8/RConn2 -- Branch8-8/RConn3 -- B-GND12/LConn1
  Branch9-9/RConn1 -- Branch9-9/RConn2 -- Branch9-9/RConn3 -- B-GND14/LConn1
  Branch10-10/RConn1 -- Branch10-10/RConn2 -- Branch10-10/RConn3 -- B-GND17/LConn1
  Branch11-11/RConn1 -- Branch11-11/RConn2 -- Branch11-11/RConn3 -- B-GND19/LConn1
  Branch12-12/RConn1 -- Branch12-12/RConn2 -- Branch12-12/RConn3 -- B-GND23/LConn1
  Branch13-13/RConn1 -- Branch13-13/RConn2 -- Branch13-13/RConn3 -- B-GND26/LConn1
  Branch14-14/RConn1 -- Branch14-14/RConn2 -- Branch14-14/RConn3 -- B-GND29/LConn1
  Branch15-15/RConn1 -- Branch15-15/RConn2 -- Branch15-15/RConn3 -- B-GND32/LConn1
  Branch16-16/RConn1 -- Branch16-16/RConn2 -- Branch16-16/RConn3 -- B-GND35/LConn1
  Branch17-17/RConn1 -- Branch17-17/RConn2 -- Branch17-17/RConn3 -- B-GND37/LConn1
  Branch18-18/RConn1 -- Branch18-18/RConn2 -- Branch18-18/RConn3 -- B-GND39/LConn1
  Branch19-19/RConn1 -- Branch19-19/RConn2 -- Branch19-19/RConn3 -- B-GND40/LConn1
  Branch20-20/RConn1 -- Branch20-20/RConn2 -- Branch20-20/RConn3 -- B-GND43/LConn1
  Branch21-21/RConn1 -- Branch21-21/RConn2 -- Branch21-21/RConn3 -- B-GND45/LConn1
  Branch22-22/RConn1 -- Branch22-22/RConn2 -- Branch22-22/RConn3 -- B-GND47/LConn1
  Branch23-23/RConn1 -- Branch23-23/RConn2 -- Branch23-23/RConn3 -- B-GND49/LConn1
  Branch24-24/RConn1 -- Branch24-24/RConn2 -- Branch24-24/RConn3 -- B-GND51/LConn1
  Branch25-25/RConn1 -- Branch25-25/RConn2 -- Branch25-25/RConn3 -- B-GND53/LConn1
  Branch26-26/RConn1 -- Branch26-26/RConn2 -- Branch26-26/RConn3 -- B-GND58/LConn1
  Branch27-27/RConn1 -- Branch27-27/RConn2 -- Branch27-27/RConn3 -- B-GND61/LConn1
  Branch28-28/RConn1 -- Branch28-28/RConn2 -- Branch28-28/RConn3 -- B-GND62/LConn1
  Branch29-29/RConn1 -- Branch29-29/RConn2 -- Branch29-29/RConn3 -- B-GND64/LConn1
  Branch30-30/RConn1 -- Branch30-30/RConn2 -- Branch30-30/RConn3 -- B-GND65/LConn1
  Branch31-31/RConn1 -- Branch31-31/RConn2 -- Branch31-31/RConn3 -- B-GND67/LConn1
  Branch32-32/RConn1 -- Branch32-32/RConn2 -- Branch32-32/RConn3 -- B-GND69/LConn1
  Branch33-33/RConn1 -- Branch33-33/RConn2 -- Branch33-33/RConn3 -- B-GND71/LConn1
  Branch34-34/RConn1 -- Branch34-34/RConn2 -- Branch34-34/RConn3 -- B-GND72/LConn1
  Branch35-35/RConn1 -- Branch35-35/RConn2 -- Branch35-35/RConn3 -- B-GND74/LConn1
  Branch36-36/RConn1 -- Branch36-36/RConn2 -- Branch36-36/RConn3 -- B-GND78/LConn1
  Branch37-37/RConn1 -- Branch37-37/RConn2 -- Branch37-37/RConn3 -- B-GND79/LConn1
  Branch38-38/RConn1 -- Branch38-38/RConn2 -- Branch38-38/RConn3 -- B-GND81/LConn1
  Branch39-39/RConn1 -- Branch39-39/RConn2 -- Branch39-39/RConn3 -- B-GND82/LConn1
  Branch1-32/RConn1 -- Bus32/RConn1 -- Branch32-32/LConn1 -- Branch32-33/LConn1 -- Branch31-32/RConn1
  Branch1-32/RConn2 -- Bus32/RConn2 -- Branch32-32/LConn2 -- Branch32-33/LConn2 -- Branch31-32/RConn2
  Branch1-32/RConn3 -- Bus32/RConn3 -- Branch32-32/LConn3 -- Branch32-33/LConn3 -- Branch31-32/RConn3
  Bus1/RConn1 -- Branch1-32/LConn1
  Bus1/RConn2 -- Branch1-32/LConn2
  Bus1/RConn3 -- Branch1-32/LConn3
  Branch2-15/RConn1 -- Bus15/RConn1 -- Branch15-15/LConn1 -- Branch15-20/LConn1 -- Branch15-16/LConn1 -- Branch14-15/RConn1
  Branch2-15/RConn2 -- Bus15/RConn2 -- Branch15-15/LConn2 -- Branch15-20/LConn2 -- Branch15-16/LConn2 -- Branch14-15/RConn2
  Branch2-15/RConn3 -- Bus15/RConn3 -- Branch15-15/LConn3 -- Branch15-20/LConn3 -- Branch15-16/LConn3 -- Branch14-15/RConn3
  Branch2-15/LConn1 -- Bus2/RConn1 -- Branch2-2/LConn1
  Branch2-15/LConn2 -- Bus2/RConn2 -- Branch2-2/LConn2
  Branch2-15/LConn3 -- Bus2/RConn3 -- Branch2-2/LConn3
  Branch3-19/RConn1 -- Bus19/RConn1 -- Branch19-19/LConn1 -- Branch19-22/LConn1 -- Branch19-20/LConn1
  Branch3-19/RConn2 -- Bus19/RConn2 -- Branch19-19/LConn2 -- Branch19-22/LConn2 -- Branch19-20/LConn2
  Branch3-19/RConn3 -- Bus19/RConn3 -- Branch19-19/LConn3 -- Branch19-22/LConn3 -- Branch19-20/LConn3
  Branch3-19/LConn1 -- Bus3/RConn1 -- Branch3-3/LConn1
  Branch3-19/LConn2 -- Bus3/RConn2 -- Branch3-3/LConn2
  Branch3-19/LConn3 -- Bus3/RConn3 -- Branch3-3/LConn3
  Branch4-28/RConn1 -- Bus28/RConn1 -- Branch28-28/LConn1 -- Branch28-29/LConn1 -- Branch25-28/RConn1
  Branch4-28/RConn2 -- Bus28/RConn2 -- Branch28-28/LConn2 -- Branch28-29/LConn2 -- Branch25-28/RConn2
  Branch4-28/RConn3 -- Bus28/RConn3 -- Branch28-28/LConn3 -- Branch28-29/LConn3 -- Branch25-28/RConn3
  Bus4/RConn1 -- Branch4-28/LConn1
  Bus4/RConn2 -- Branch4-28/LConn2
  Bus4/RConn3 -- Branch4-28/LConn3
  Branch5-29/RConn1 -- Bus29/RConn1 -- Branch29-29/LConn1 -- Branch28-29/RConn1
  Branch5-29/RConn2 -- Bus29/RConn2 -- Branch29-29/LConn2 -- Branch28-29/RConn2
  Branch5-29/RConn3 -- Bus29/RConn3 -- Branch29-29/LConn3 -- Branch28-29/RConn3
  Branch5-29/LConn1 -- Bus5/RConn1 -- Branch5-5/LConn1
  Branch5-29/LConn2 -- Bus5/RConn2 -- Branch5-5/LConn2
  Branch5-29/LConn3 -- Bus5/RConn3 -- Branch5-5/LConn3
  Branch6-31/RConn1 -- Bus31/RConn1 -- Branch31-31/LConn1 -- Branch31-32/LConn1 -- Branch30-31/RConn1
  Branch6-31/RConn2 -- Bus31/RConn2 -- Branch31-31/LConn2 -- Branch31-32/LConn2 -- Branch30-31/RConn2
  Branch6-31/RConn3 -- Bus31/RConn3 -- Branch31-31/LConn3 -- Branch31-32/LConn3 -- Branch30-31/RConn3
  Bus6/RConn1 -- Branch6-31/LConn1
  Bus6/RConn2 -- Branch6-31/LConn2
  Bus6/RConn3 -- Branch6-31/LConn3
  Branch7-34/RConn1 -- Bus34/RConn1 -- Branch34-34/LConn1 -- Branch34-35/LConn1 -- Branch11-34/RConn1
  Branch7-34/RConn2 -- Bus34/RConn2 -- Branch34-34/LConn2 -- Branch34-35/LConn2 -- Branch11-34/RConn2
  Branch7-34/RConn3 -- Bus34/RConn3 -- Branch34-34/LConn3 -- Branch34-35/LConn3 -- Branch11-34/RConn3
  Branch7-34/LConn1 -- Bus7/RConn1 -- Branch7-7/LConn1
  Branch7-34/LConn2 -- Bus7/RConn2 -- Branch7-7/LConn2
  Branch7-34/LConn3 -- Bus7/RConn3 -- Branch7-7/LConn3
  Branch8-38/RConn1 -- Bus38/RConn1 -- Branch38-38/LConn1 -- Branch37-38/RConn1 -- Branch35-38/RConn1
  Branch8-38/RConn2 -- Bus38/RConn2 -- Branch38-38/LConn2 -- Branch37-38/RConn2 -- Branch35-38/RConn2
  Branch8-38/RConn3 -- Bus38/RConn3 -- Branch38-38/LConn3 -- Branch37-38/RConn3 -- Branch35-38/RConn3
  Branch8-38/LConn1 -- Bus8/RConn1 -- Branch8-8/LConn1
  Branch8-38/LConn2 -- Bus8/RConn2 -- Branch8-8/LConn2
  Branch8-38/LConn3 -- Bus8/RConn3 -- Branch8-8/LConn3
  Branch9-10/RConn1 -- Bus10/RConn1 -- Branch10-10/LConn1 -- Branch10-11/LConn1
  Branch9-10/RConn2 -- Bus10/RConn2 -- Branch10-10/LConn2 -- Branch10-11/LConn2
  Branch9-10/RConn3 -- Bus10/RConn3 -- Branch10-10/LConn3 -- Branch10-11/LConn3
  Branch9-10/LConn1 -- Bus9/RConn1 -- Branch9-9/LConn1 -- Branch9-18/LConn1
  Branch9-10/LConn2 -- Bus9/RConn2 -- Branch9-9/LConn2 -- Branch9-18/LConn2
  Branch9-10/LConn3 -- Bus9/RConn3 -- Branch9-9/LConn3 -- Branch9-18/LConn3
  Branch9-18/RConn1 -- Bus18/RConn1 -- Branch18-18/LConn1 -- Branch17-18/RConn1
  Branch9-18/RConn2 -- Bus18/RConn2 -- Branch18-18/LConn2 -- Branch17-18/RConn2
  Branch9-18/RConn3 -- Bus18/RConn3 -- Branch18-18/LConn3 -- Branch17-18/RConn3
  Branch10-11/RConn1 -- Bus11/RConn1 -- Branch11-11/LConn1 -- Branch11-39/LConn1 -- Branch11-34/LConn1 -- Branch11-12/LConn1
  Branch10-11/RConn2 -- Bus11/RConn2 -- Branch11-11/LConn2 -- Branch11-39/LConn2 -- Branch11-34/LConn2 -- Branch11-12/LConn2
  Branch10-11/RConn3 -- Bus11/RConn3 -- Branch11-11/LConn3 -- Branch11-39/LConn3 -- Branch11-34/LConn3 -- Branch11-12/LConn3
  Branch11-12/RConn1 -- Bus12/RConn1 -- Branch12-12/LConn1 -- Branch12-27/LConn1 -- Branch12-13/LConn1
  Branch11-12/RConn2 -- Bus12/RConn2 -- Branch12-12/LConn2 -- Branch12-27/LConn2 -- Branch12-13/LConn2
  Branch11-12/RConn3 -- Bus12/RConn3 -- Branch12-12/LConn3 -- Branch12-27/LConn3 -- Branch12-13/LConn3
  Branch11-39/RConn1 -- Bus39/RConn1 -- Branch39-39/LConn1
  Branch11-39/RConn2 -- Bus39/RConn2 -- Branch39-39/LConn2
  Branch11-39/RConn3 -- Bus39/RConn3 -- Branch39-39/LConn3
  Branch12-13/RConn1 -- Bus13/RConn1 -- Branch13-13/LConn1 -- Branch13-23/LConn1 -- Branch13-14/LConn1
  Branch12-13/RConn2 -- Bus13/RConn2 -- Branch13-13/LConn2 -- Branch13-23/LConn2 -- Branch13-14/LConn2
  Branch12-13/RConn3 -- Bus13/RConn3 -- Branch13-13/LConn3 -- Branch13-23/LConn3 -- Branch13-14/LConn3
  Branch12-27/RConn1 -- Bus27/RConn1 -- Branch27-27/LConn1 -- Branch26-27/RConn1
  Branch12-27/RConn2 -- Bus27/RConn2 -- Branch27-27/LConn2 -- Branch26-27/RConn2
  Branch12-27/RConn3 -- Bus27/RConn3 -- Branch27-27/LConn3 -- Branch26-27/RConn3
  Branch13-14/RConn1 -- Bus14/RConn1 -- Branch14-14/LConn1 -- Branch14-17/LConn1 -- Branch14-15/LConn1
  Branch13-14/RConn2 -- Bus14/RConn2 -- Branch14-14/LConn2 -- Branch14-17/LConn2 -- Branch14-15/LConn2
  Branch13-14/RConn3 -- Bus14/RConn3 -- Branch14-14/LConn3 -- Branch14-17/LConn3 -- Branch14-15/LConn3
  Branch13-23/RConn1 -- Bus23/RConn1 -- Branch23-23/LConn1 -- Branch23-24/LConn1 -- Branch22-23/RConn1
  Branch13-23/RConn2 -- Bus23/RConn2 -- Branch23-23/LConn2 -- Branch23-24/LConn2 -- Branch22-23/RConn2
  Branch13-23/RConn3 -- Bus23/RConn3 -- Branch23-23/LConn3 -- Branch23-24/LConn3 -- Branch22-23/RConn3
  Branch14-17/RConn1 -- Bus17/RConn1 -- Branch17-17/LConn1 -- Branch17-18/LConn1 -- Branch16-17/RConn1
  Branch14-17/RConn2 -- Bus17/RConn2 -- Branch17-17/LConn2 -- Branch17-18/LConn2 -- Branch16-17/RConn2
  Branch14-17/RConn3 -- Bus17/RConn3 -- Branch17-17/LConn3 -- Branch17-18/LConn3 -- Branch16-17/RConn3
  Branch15-16/RConn1 -- Bus16/RConn1 -- Branch16-16/LConn1 -- Branch16-17/LConn1
  Branch15-16/RConn2 -- Bus16/RConn2 -- Branch16-16/LConn2 -- Branch16-17/LConn2
  Branch15-16/RConn3 -- Bus16/RConn3 -- Branch16-16/LConn3 -- Branch16-17/LConn3
  Branch15-20/RConn1 -- Bus20/RConn1 -- Branch20-20/LConn1 -- Branch20-21/LConn1 -- Branch19-20/RConn1
  Branch15-20/RConn2 -- Bus20/RConn2 -- Branch20-20/LConn2 -- Branch20-21/LConn2 -- Branch19-20/RConn2
  Branch15-20/RConn3 -- Bus20/RConn3 -- Branch20-20/LConn3 -- Branch20-21/LConn3 -- Branch19-20/RConn3
  Branch19-22/RConn1 -- Bus22/RConn1 -- Branch22-22/LConn1 -- Branch22-23/LConn1 -- Branch21-22/RConn1
  Branch19-22/RConn2 -- Bus22/RConn2 -- Branch22-22/LConn2 -- Branch22-23/LConn2 -- Branch21-22/RConn2
  Branch19-22/RConn3 -- Bus22/RConn3 -- Branch22-22/LConn3 -- Branch22-23/LConn3 -- Branch21-22/RConn3
  Branch20-21/RConn1 -- Bus21/RConn1 -- Branch21-21/LConn1 -- Branch21-22/LConn1
  Branch20-21/RConn2 -- Bus21/RConn2 -- Branch21-21/LConn2 -- Branch21-22/LConn2
  Branch20-21/RConn3 -- Bus21/RConn3 -- Branch21-21/LConn3 -- Branch21-22/LConn3
  Branch23-24/RConn1 -- Bus24/RConn1 -- Branch24-24/LConn1 -- Branch24-25/LConn1
  Branch23-24/RConn2 -- Bus24/RConn2 -- Branch24-24/LConn2 -- Branch24-25/LConn2
  Branch23-24/RConn3 -- Bus24/RConn3 -- Branch24-24/LConn3 -- Branch24-25/LConn3
  Branch24-25/RConn1 -- Bus25/RConn1 -- Branch25-25/LConn1 -- Branch25-33/LConn1 -- Branch25-30/LConn1 -- Branch25-28/LConn1 -- Branch25-26/LConn1
  Branch24-25/RConn2 -- Bus25/RConn2 -- Branch25-25/LConn2 -- Branch25-33/LConn2 -- Branch25-30/LConn2 -- Branch25-28/LConn2 -- Branch25-26/LConn2
  Branch24-25/RConn3 -- Bus25/RConn3 -- Branch25-25/LConn3 -- Branch25-33/LConn3 -- Branch25-30/LConn3 -- Branch25-28/LConn3 -- Branch25-26/LConn3
  Branch25-26/RConn1 -- Bus26/RConn1 -- Branch26-26/LConn1 -- Branch26-36/LConn1 -- Branch26-27/LConn1
  Branch25-26/RConn2 -- Bus26/RConn2 -- Branch26-26/LConn2 -- Branch26-36/LConn2 -- Branch26-27/LConn2
  Branch25-26/RConn3 -- Bus26/RConn3 -- Branch26-26/LConn3 -- Branch26-36/LConn3 -- Branch26-27/LConn3
  Branch25-30/RConn1 -- Bus30/RConn1 -- Branch30-30/LConn1 -- Branch30-31/LConn1
  Branch25-30/RConn2 -- Bus30/RConn2 -- Branch30-30/LConn2 -- Branch30-31/LConn2
  Branch25-30/RConn3 -- Bus30/RConn3 -- Branch30-30/LConn3 -- Branch30-31/LConn3
  Branch25-33/RConn1 -- Bus33/RConn1 -- Branch33-33/LConn1 -- Branch32-33/RConn1
  Branch25-33/RConn2 -- Bus33/RConn2 -- Branch33-33/LConn2 -- Branch32-33/RConn2
  Branch25-33/RConn3 -- Bus33/RConn3 -- Branch33-33/LConn3 -- Branch32-33/RConn3
  Branch26-36/RConn1 -- Bus36/RConn1 -- Branch36-36/LConn1 -- Branch35-36/RConn1
  Branch26-36/RConn2 -- Bus36/RConn2 -- Branch36-36/LConn2 -- Branch35-36/RConn2
  Branch26-36/RConn3 -- Bus36/RConn3 -- Branch36-36/LConn3 -- Branch35-36/RConn3
  Branch34-35/RConn1 -- Bus35/RConn1 -- Branch35-35/LConn1 -- Branch35-38/LConn1 -- Branch35-37/LConn1 -- Branch35-36/LConn1
  Branch34-35/RConn2 -- Bus35/RConn2 -- Branch35-35/LConn2 -- Branch35-38/LConn2 -- Branch35-37/LConn2 -- Branch35-36/LConn2
  Branch34-35/RConn3 -- Bus35/RConn3 -- Branch35-35/LConn3 -- Branch35-38/LConn3 -- Branch35-37/LConn3 -- Branch35-36/LConn3
  Branch35-37/RConn1 -- Bus37/RConn1 -- Branch37-37/LConn1 -- Branch37-38/LConn1
  Branch35-37/RConn2 -- Bus37/RConn2 -- Branch37-37/LConn2 -- Branch37-38/LConn2
  Branch35-37/RConn3 -- Bus37/RConn3 -- Branch37-37/LConn3 -- Branch37-38/LConn3
  Inf-Bus1/LConn1 -- Bus1/LConn1
  Inf-Bus1/LConn2 -- Bus1/LConn2
  Inf-Bus1/LConn3 -- Bus1/LConn3
  VSI-PLL2/LConn1 -- Bus2/LConn1
  VSI-PLL2/LConn2 -- Bus2/LConn2
  VSI-PLL2/LConn3 -- Bus2/LConn3
  VSI-PLL3/LConn1 -- Bus3/LConn1
  VSI-PLL3/LConn2 -- Bus3/LConn2
  VSI-PLL3/LConn3 -- Bus3/LConn3
  VSI-Droop4/LConn1 -- Bus4/LConn1
  VSI-Droop4/LConn2 -- Bus4/LConn2
  VSI-Droop4/LConn3 -- Bus4/LConn3
  VSI-PLL5/LConn1 -- Bus5/LConn1
  VSI-PLL5/LConn2 -- Bus5/LConn2
  VSI-PLL5/LConn3 -- Bus5/LConn3
  VSI-Droop6/LConn1 -- Bus6/LConn1
  VSI-Droop6/LConn2 -- Bus6/LConn2
  VSI-Droop6/LConn3 -- Bus6/LConn3
  VSI-PLL7/LConn1 -- Bus7/LConn1
  VSI-PLL7/LConn2 -- Bus7/LConn2
  VSI-PLL7/LConn3 -- Bus7/LConn3
  VSI-PLL8/LConn1 -- Bus8/LConn1
  VSI-PLL8/LConn2 -- Bus8/LConn2
  VSI-PLL8/LConn3 -- Bus8/LConn3
  VSI-PLL9/LConn1 -- Bus9/LConn1
  VSI-PLL9/LConn2 -- Bus9/LConn2
  VSI-PLL9/LConn3 -- Bus9/LConn3
  VSI-PLL10/LConn1 -- Bus10/LConn1
  VSI-PLL10/LConn2 -- Bus10/LConn2
  VSI-PLL10/LConn3 -- Bus10/LConn3
  VSI-PLL11/LConn1 -- Bus11/LConn1
  VSI-PLL11/LConn2 -- Bus11/LConn2
  VSI-PLL11/LConn3 -- Bus11/LConn3
  VSI-PLL39/LConn1 -- Bus39/LConn1
  VSI-PLL39/LConn2 -- Bus39/LConn2
  VSI-PLL39/LConn3 -- Bus39/LConn3
